simulink model "temperature"  (R2018b)
settings: Solver=FixedStepAuto  StartTime=1  StopTime=intervals  FixedStep=1  RelTol=1e-3
values from neighbouring files (symbols this model uses):
  stepsInDay = 24*60/timeStep    (= 288)    [init.m]
  sunrise = floor(0.25*stepsInDay)    [init.m]
  sunset = floor(0.8*stepsInDay)    [init.m]
settings Model: EnablePacing=on  PacingRate=10  Creator=rexlu  LastModifiedBy=hans

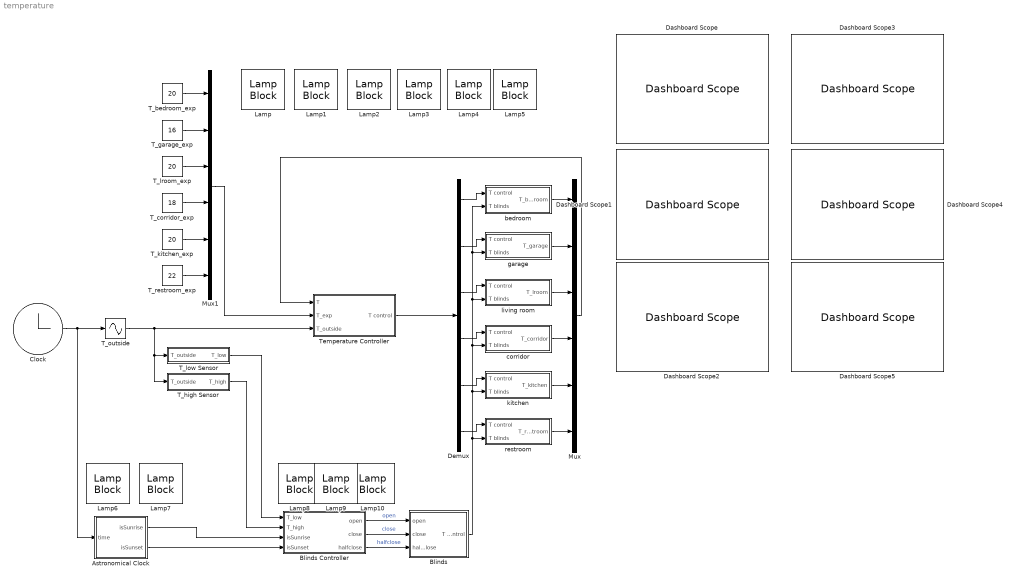
== system temperature ==
  Astronomical Clock : Subsystem
  Blinds : Subsystem
  Blinds Controller : Stateflow chart  TreatAsAtomicUnit=on
  "Clock " : Clock
  Dashboard Scope : DashboardScope  WebBlockId=186
  Dashboard Scope1 : DashboardScope  WebBlockId=187
  Dashboard Scope2 : DashboardScope  WebBlockId=188
  Dashboard Scope3 : DashboardScope  WebBlockId=189
  Dashboard Scope4 : DashboardScope  WebBlockId=190
  Dashboard Scope5 : DashboardScope  WebBlockId=191
  Demux : Demux  Outputs=6
  Lamp : LampBlock  WebBlockId=33
  Lamp1 : LampBlock  WebBlockId=181
  Lamp10 : LampBlock  WebBlockId=261
  Lamp2 : LampBlock  WebBlockId=182
  Lamp3 : LampBlock  WebBlockId=183
  Lamp4 : LampBlock  WebBlockId=184
  Lamp5 : LampBlock  WebBlockId=185
  Lamp6 : LampBlock  WebBlockId=198
  Lamp7 : LampBlock  WebBlockId=199
  Lamp8 : LampBlock  WebBlockId=259
  Lamp9 : LampBlock  WebBlockId=260
  Mux : Mux  Inputs=6
  Mux1 : Mux  Inputs=6
  T_bedroom_exp : Constant  Value=20
  T_corridor_exp : Constant  Value=18
  T_garage_exp : Constant  Value=16
  T_high Sensor : Subsystem
  T_kitchen_exp : Constant  Value=20
  T_low Sensor : Subsystem
  T_lroom_exp : Constant  Value=20
  T_outside : Sin  TimeSource=Use external signal  Amplitude=18  Bias=10  Frequency=2*pi/stepsInDay  Phase=-pi/2  SampleTime=0
  T_restroom_exp : Constant  Value=22
  Temperature Controller : Subsystem
  bedroom : Subsystem
  corridor : Subsystem
  garage : Subsystem
  kitchen : Subsystem
  living room : Subsystem
  restroom : Subsystem
  wires:
  "Clock "/1 -> Astronomical Clock/1(time), T_outside/1
  bedroom/1(T_bedroom) -> Mux/1
  garage/1(T_garage) -> Mux/2
  living room/1(T_lroom) -> Mux/3
  corridor/1(T_corridor) -> Mux/4
  kitchen/1(T_kitchen) -> Mux/5
  restroom/1(T_restroom) -> Mux/6
  Mux/1 -> Temperature Controller/1(T)
  Demux/1 -> bedroom/1(T control)
  Demux/2 -> garage/1(T control)
  Demux/3 -> living room/1(T control)
  Demux/4 -> corridor/1(T control)
  Demux/5 -> kitchen/1(T control)
  Demux/6 -> restroom/1(T control)
  T_bedroom_exp/1 -> Mux1/1
  T_garage_exp/1 -> Mux1/2
  T_lroom_exp/1 -> Mux1/3
  T_corridor_exp/1 -> Mux1/4
  T_kitchen_exp/1 -> Mux1/5
  T_restroom_exp/1 -> Mux1/6
  Mux1/1 -> Temperature Controller/2(T_exp)
  T_outside/1 -> T_high Sensor/1(T_outside), T_low Sensor/1(T_outside), Temperature Controller/3(T_outside)
  Astronomical Clock/1(isSunrise) -> Blinds Controller/3(isSunrise)
  Astronomical Clock/2(isSunset) -> Blinds Controller/4(isSunset)
  Temperature Controller/1(T control) -> Demux/1
  T_low Sensor/1(T_low) -> Blinds Controller/1(T_low)
  T_high Sensor/1(T_high) -> Blinds Controller/2(T_high)
  Blinds Controller/1(open) -> Blinds/1(open)  "open"
  Blinds Controller/2(close) -> Blinds/2(close)  "close"
  Blinds Controller/3(halfclose) -> Blinds/3(halfclose)  "halfclose"
  Blinds/1(T control) -> bedroom/2(T blinds), garage/2(T blinds), living room/2(T blinds), corridor/2(T blinds), kitchen/2(T blinds), restroom/2(T blinds)

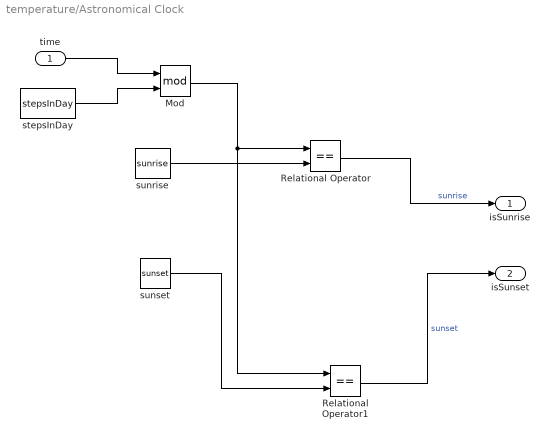
== system temperature/Astronomical Clock ==
  time : Inport
  Mod : Math  Operator=mod  SaturateOnIntegerOverflow=on
  Relational Operator : RelationalOperator  Operator===  OutDataTypeStr=boolean  RndMeth=Simplest
  Relational Operator1 : RelationalOperator  Operator===  OutDataTypeStr=boolean  RndMeth=Simplest
  stepsInDay : Constant  Value=stepsInDay
  sunrise : Constant  Value=sunrise
  sunset : Constant  Value=sunset
  isSunrise : Outport
  isSunset : Outport  Port=2
  wires:
  Relational Operator1/1 -> isSunset/1  "sunset"
  sunrise/1 -> Relational Operator/2
  Relational Operator/1 -> isSunrise/1  "sunrise"
  sunset/1 -> Relational Operator1/2
  time/1 -> Mod/1
  Mod/1 -> Relational Operator1/1, Relational Operator/1
  stepsInDay/1 -> Mod/2

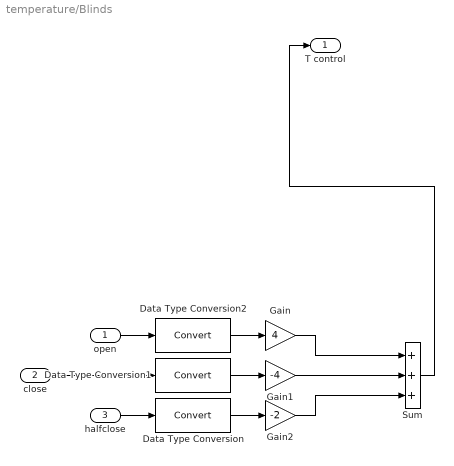
== system temperature/Blinds ==
  open : Inport
  close : Inport  Port=2
  halfclose : Inport  Port=3
  Data Type Conversion : DataTypeConversion
  Data Type Conversion1 : DataTypeConversion
  Data Type Conversion2 : DataTypeConversion
  Gain : Gain  Gain=4
  Gain1 : Gain  Gain=-4
  Gain2 : Gain  Gain=-2
  Sum : Sum  Inputs=+++
  T control : Outport
  wires:
  Gain/1 -> Sum/1
  halfclose/1 -> Data Type Conversion/1
  Gain1/1 -> Sum/2
  close/1 -> Data Type Conversion1/1
  Gain2/1 -> Sum/3
  open/1 -> Data Type Conversion2/1
  Sum/1 -> T control/1
  Data Type Conversion/1 -> Gain2/1
  Data Type Conversion1/1 -> Gain1/1
  Data Type Conversion2/1 -> Gain/1

== system temperature/T_high Sensor ==
  T_outside : Inport
  Relational Operator : RelationalOperator  Operator=>  OutDataTypeStr=boolean  RndMeth=Simplest
  T_cap_H : Constant  Value=25
  T_high : Outport
  wires:
  T_outside/1 -> Relational Operator/1
  T_cap_H/1 -> Relational Operator/2
  Relational Operator/1 -> T_high/1  "T_cap_H"

== system temperature/T_low Sensor ==
  T_outside : Inport
  Relational Operator1 : RelationalOperator  Operator=<  OutDataTypeStr=boolean  RndMeth=Simplest
  T_cap_L : Constant  Value=-5
  T_low : Outport
  wires:
  T_cap_L/1 -> Relational Operator1/2
  Relational Operator1/1 -> T_low/1  "T_cap_L"
  T_outside/1 -> Relational Operator1/1

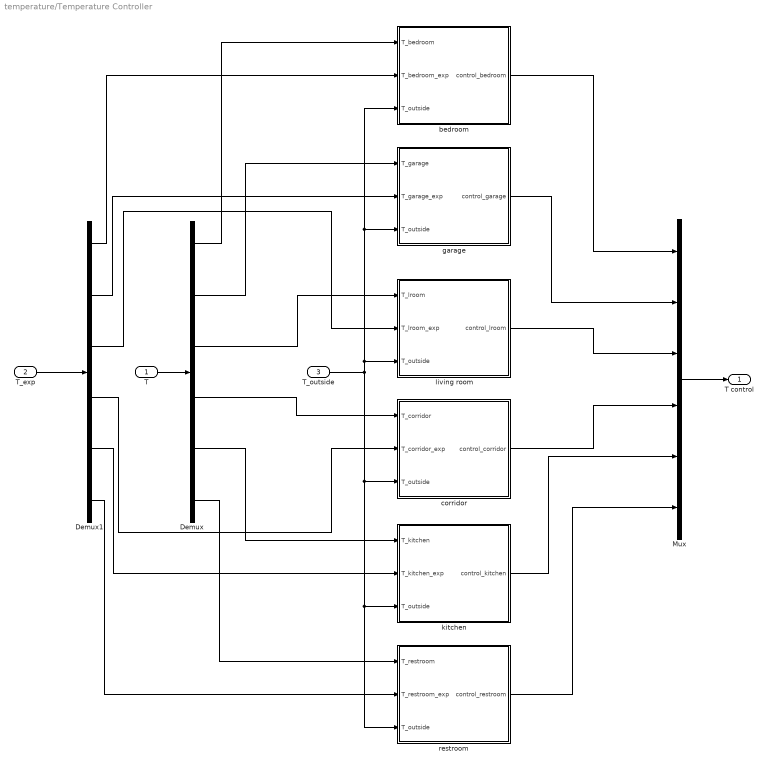
== system temperature/Temperature Controller ==
  T : Inport
  T_exp : Inport  Port=2
  T_outside : Inport  Port=3
  Demux : Demux  Outputs=6
  Demux1 : Demux  Outputs=6
  Mux : Mux  Inputs=6
  bedroom : Subsystem
  corridor : Subsystem
  garage : Subsystem
  kitchen : Subsystem
  living room : Subsystem
  restroom : Subsystem
  T control : Outport
  wires:
  T/1 -> Demux/1
  T_exp/1 -> Demux1/1
  Demux/1 -> bedroom/1(T_bedroom)
  Demux/2 -> garage/1(T_garage)
  Demux/3 -> living room/1(T_lroom)
  Demux/4 -> corridor/1(T_corridor)
  Demux/5 -> kitchen/1(T_kitchen)
  Demux/6 -> restroom/1(T_restroom)
  Demux1/1 -> bedroom/2(T_bedroom_exp)
  Demux1/2 -> garage/2(T_garage_exp)
  Demux1/3 -> living room/2(T_lroom_exp)
  Demux1/4 -> corridor/2(T_corridor_exp)
  Demux1/5 -> kitchen/2(T_kitchen_exp)
  Demux1/6 -> restroom/2(T_restroom_exp)
  bedroom/1(control_bedroom) -> Mux/1
  garage/1(control_garage) -> Mux/2
  living room/1(control_lroom) -> Mux/3
  corridor/1(control_corridor) -> Mux/4
  kitchen/1(control_kitchen) -> Mux/5
  restroom/1(control_restroom) -> Mux/6
  Mux/1 -> T control/1
  T_outside/1 -> living room/3(T_outside), bedroom/3(T_outside), garage/3(T_outside), restroom/3(T_outside), kitchen/3(T_outside), corridor/3(T_outside)

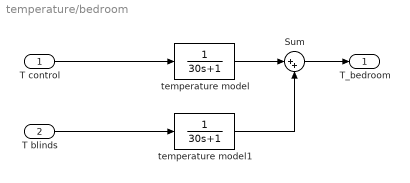
== system temperature/bedroom ==
  T control : Inport
  T blinds : Inport  Port=2
  Sum : Sum  Inputs=|++
  temperature model : TransferFcn  Denominator=[30 1]
  temperature model1 : TransferFcn  Denominator=[30 1]
  T_bedroom : Outport
  wires:
  T control/1 -> temperature model/1
  T blinds/1 -> temperature model1/1
  temperature model/1 -> Sum/1
  Sum/1 -> T_bedroom/1
  temperature model1/1 -> Sum/2

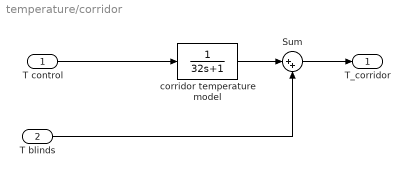
== system temperature/corridor ==
  T control : Inport
  T blinds : Inport  Port=2
  Sum : Sum  Inputs=|++
  corridor temperature model : TransferFcn  Denominator=[32 1]
  T_corridor : Outport
  wires:
  corridor temperature model/1 -> Sum/1
  T control/1 -> corridor temperature model/1
  T blinds/1 -> Sum/2
  Sum/1 -> T_corridor/1

== system temperature/garage ==
  T control : Inport
  T blinds : Inport  Port=2
  Sum : Sum  Inputs=|++
  temperature model : TransferFcn  Denominator=[18 1]
  T_garage : Outport
  wires:
  T control/1 -> temperature model/1
  T blinds/1 -> Sum/2
  temperature model/1 -> Sum/1
  Sum/1 -> T_garage/1

== system temperature/kitchen ==
  T control : Inport
  T blinds : Inport  Port=2
  Sum : Sum  Inputs=|++
  kitchen temperature model : TransferFcn  Denominator=[32 1]
  T_kitchen : Outport
  wires:
  kitchen temperature model/1 -> Sum/1
  T control/1 -> kitchen temperature model/1
  T blinds/1 -> Sum/2
  Sum/1 -> T_kitchen/1

== system temperature/living room ==
  T control : Inport
  T blinds : Inport  Port=2
  Sum : Sum  Inputs=|++
  living room temperature model : TransferFcn  Denominator=[25 1]
  T_lroom : Outport
  wires:
  T control/1 -> living room temperature model/1
  T blinds/1 -> Sum/2
  living room temperature model/1 -> Sum/1
  Sum/1 -> T_lroom/1

== system temperature/restroom ==
  T control : Inport
  T blinds : Inport  Port=2
  Sum : Sum  Inputs=|++
  restroom temperature model : TransferFcn  Denominator=[32 1]
  T_restroom : Outport
  wires:
  restroom temperature model/1 -> Sum/1
  T control/1 -> restroom temperature model/1
  T blinds/1 -> Sum/2
  Sum/1 -> T_restroom/1

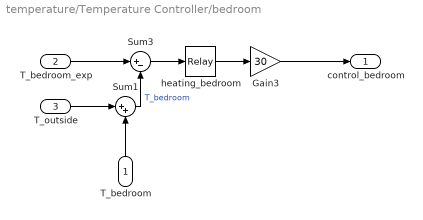
== system temperature/Temperature Controller/bedroom ==
  T_bedroom : Inport
  T_bedroom_exp : Inport  Port=2
  T_outside : Inport  Port=3
  Gain3 : Gain  Gain=30
  Sum1 : Sum  Inputs=|++
  Sum3 : Sum  Inputs=|+-
  heating_bedroom : Relay  OnSwitchValue=2  OffSwitchValue=-2
  control_bedroom : Outport
  wires:
  T_bedroom_exp/1 -> Sum3/1
  Sum1/1 -> Sum3/2  "T_bedroom"
  Gain3/1 -> control_bedroom/1
  T_bedroom/1 -> Sum1/2
  Sum3/1 -> heating_bedroom/1
  heating_bedroom/1 -> Gain3/1
  T_outside/1 -> Sum1/1

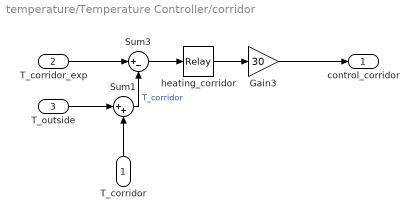
== system temperature/Temperature Controller/corridor ==
  T_corridor : Inport
  T_corridor_exp : Inport  Port=2
  T_outside : Inport  Port=3
  Gain3 : Gain  Gain=30
  Sum1 : Sum  Inputs=|++
  Sum3 : Sum  Inputs=|+-
  heating_corridor : Relay  OnSwitchValue=2  OffSwitchValue=-2
  control_corridor : Outport
  wires:
  T_corridor_exp/1 -> Sum3/1
  Sum1/1 -> Sum3/2  "T_corridor"
  Gain3/1 -> control_corridor/1
  T_corridor/1 -> Sum1/2
  Sum3/1 -> heating_corridor/1
  heating_corridor/1 -> Gain3/1
  T_outside/1 -> Sum1/1

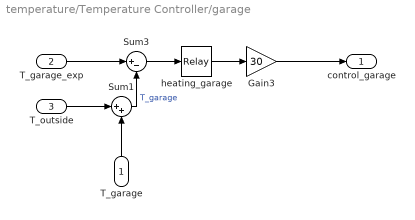
== system temperature/Temperature Controller/garage ==
  T_garage : Inport
  T_garage_exp : Inport  Port=2
  T_outside : Inport  Port=3
  Gain3 : Gain  Gain=30
  Sum1 : Sum  Inputs=|++
  Sum3 : Sum  Inputs=|+-
  heating_garage : Relay  OnSwitchValue=2  OffSwitchValue=-2
  control_garage : Outport
  wires:
  T_garage_exp/1 -> Sum3/1
  Sum1/1 -> Sum3/2  "T_garage"
  Gain3/1 -> control_garage/1
  T_garage/1 -> Sum1/2
  Sum3/1 -> heating_garage/1
  heating_garage/1 -> Gain3/1
  T_outside/1 -> Sum1/1

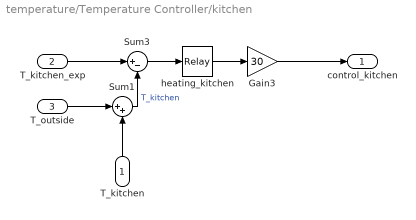
== system temperature/Temperature Controller/kitchen ==
  T_kitchen : Inport
  T_kitchen_exp : Inport  Port=2
  T_outside : Inport  Port=3
  Gain3 : Gain  Gain=30
  Sum1 : Sum  Inputs=|++
  Sum3 : Sum  Inputs=|+-
  heating_kitchen : Relay  OnSwitchValue=2  OffSwitchValue=-2
  control_kitchen : Outport
  wires:
  T_kitchen_exp/1 -> Sum3/1
  Sum1/1 -> Sum3/2  "T_kitchen"
  Gain3/1 -> control_kitchen/1
  T_kitchen/1 -> Sum1/2
  Sum3/1 -> heating_kitchen/1
  heating_kitchen/1 -> Gain3/1
  T_outside/1 -> Sum1/1

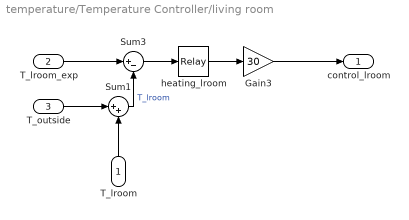
== system temperature/Temperature Controller/living room ==
  T_lroom : Inport
  T_lroom_exp : Inport  Port=2
  T_outside : Inport  Port=3
  Gain3 : Gain  Gain=30
  Sum1 : Sum  Inputs=|++
  Sum3 : Sum  Inputs=|+-
  heating_lroom : Relay  OnSwitchValue=2  OffSwitchValue=-2
  control_lroom : Outport
  wires:
  T_lroom_exp/1 -> Sum3/1
  Sum1/1 -> Sum3/2  "T_lroom"
  Gain3/1 -> control_lroom/1
  T_lroom/1 -> Sum1/2
  Sum3/1 -> heating_lroom/1
  heating_lroom/1 -> Gain3/1
  T_outside/1 -> Sum1/1

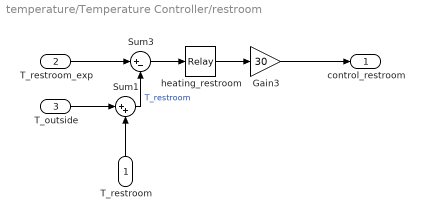
== system temperature/Temperature Controller/restroom ==
  T_restroom : Inport
  T_restroom_exp : Inport  Port=2
  T_outside : Inport  Port=3
  Gain3 : Gain  Gain=30
  Sum1 : Sum  Inputs=|++
  Sum3 : Sum  Inputs=|+-
  heating_restroom : Relay  OnSwitchValue=2  OffSwitchValue=-2
  control_restroom : Outport
  wires:
  T_restroom_exp/1 -> Sum3/1
  Sum1/1 -> Sum3/2  "T_restroom"
  Gain3/1 -> control_restroom/1
  T_restroom/1 -> Sum1/2
  Sum3/1 -> heating_restroom/1
  heating_restroom/1 -> Gain3/1
  T_outside/1 -> Sum1/1

== stateflow chart temperature/Blinds Controller ==
  settings: executeAtInitialization=1
  state State
    state HalfClose
      halfclose = true;
      open = false;
      close = false;
    state Close
      close = true;
      open = false;
      halfclose = false;
    state Open
      open = true;
      halfclose = false;
      close = false;
    (default) -> Close
    Close -> HalfClose [order 2] : [T_high]
    HalfClose -> Close [order 2] : [isSunset]
    HalfClose -> Open [order 1] : [isSunrise || T_low]
    Open -> HalfClose [order 2] : [T_high]
    Open -> Close [order 1] : [isSunset]
    Close -> Open [order 1] : [isSunrise || T_low]
  data: T_low input; T_high input; isSunrise input; isSunset input; open output boolean; close output boolean; halfclose output boolean
